simulink model "SingleAgentQUAV"  (R2018b)
settings: Solver=ode1  StartTime=0.0  StopTime=600  FixedStep=tstep  RelTol=1e-3
InitFcn:
  | initSim;
StopFcn:
  | plotSimSolution;
values from neighbouring files (symbols this model uses):
  tstep = 0.1    [initSim.m]
undefined symbols (not defined in the file or in its folder): m, problem
settings Model: Creator=yn15  LastModifiedBy=dan
settings OptimizationCC: LifeSpan=inf
settings DebuggingCC: SFUnexpectedBacktrackingDiag=warning  SFNoUnconditionalDefaultTransitionDiag=warning  SFExecutionAtInitializationDiag=none
settings SFSimCC: SimUseLocalCustomCode=off
settings RTWCC: RTWUseLocalCustomCode=off
settings CodeAppCC: StateflowObjectComments=on
settings GRTTargetCC: TargetLangStandard=C89/C90 (ANSI)
settings ConfigComp: CovMetricSettings=dw  CovHtmlReporting=on  CovSaveCumulativeToWorkspaceVar=on  CovSaveSingleToWorkspaceVar=on  CovExternalEMLEnable=off

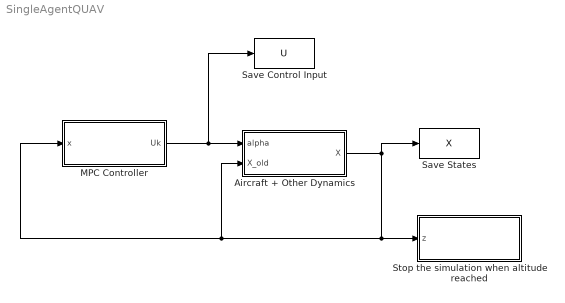
== system SingleAgentQUAV ==
  Aircraft + Other Dynamics : Subsystem
  "MPC Controller " : Subsystem
  Save Control Input : ToWorkspace  VariableName=U  SampleTime=-1
      settings: Save2DSignal=2-D array (concatenate along first dimension)
  Save States : ToWorkspace  VariableName=X  SampleTime=-1
  "Stop the simulation when altitude reached " : Subsystem
  wires:
  "MPC Controller "/1(Uk) -> Aircraft + Other Dynamics/1(alpha), Save Control Input/1
  Aircraft + Other Dynamics/1(X) -> Save States/1, "Stop the simulation when altitude reached "/1(z), Aircraft + Other Dynamics/2("X_old "), "MPC Controller "/1(x)

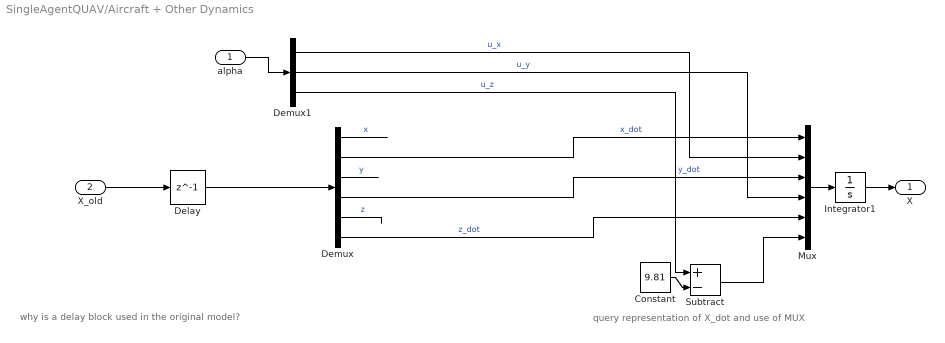
== system SingleAgentQUAV/Aircraft + Other Dynamics ==
  note: query representation of X_dot and use of MUX
  note: why is a delay block used in the original model?
  alpha : Inport
  "X_old " : Inport  Port=2
  Constant : Constant  Value=9.81
  Delay : Delay  DelayLength=1  InitialCondition=[problem.states.x0]
  Demux : Demux  Outputs=6
  Demux1 : Demux  Outputs=3
  Integrator1 : Integrator
  Mux : Mux  Inputs=6
  Subtract : Sum  Inputs=+-
  X : Outport
  wires:
  "X_old "/1 -> Delay/1
  Delay/1 -> Demux/1
  alpha/1 -> Demux1/1
  Demux/1 -> ?  "x"
  Demux/3 -> ?  "y"
  Demux/4 -> Mux/3  "y_dot"
  Demux/5 -> ?  "z"
  Demux/6 -> Mux/5  "z_dot"
  Demux1/1 -> Mux/2  "u_x"
  Demux1/2 -> Mux/4  "u_y"
  Demux1/3 -> Subtract/1  "u_z"
  Demux/2 -> Mux/1  "x_dot"
  Integrator1/1 -> X/1
  Mux/1 -> Integrator1/1
  Constant/1 -> Subtract/2
  Subtract/1 -> Mux/6

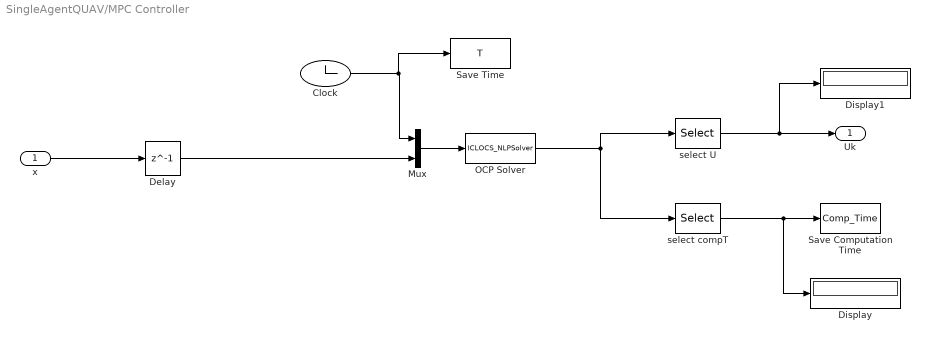
== system SingleAgentQUAV/MPC Controller  ==
  x : Inport
  Clock : Clock
  Delay : Delay  DelayLength=1  InitialCondition=[problem.states.x0]
  Display : Display
  Display1 : Display
  Mux : Mux  Inputs=2
  OCP Solver : MATLABFcn  MATLABFcn=ICLOCS_NLPSolver  OutputDimensions=m+2
  "Save Computation Time " : ToWorkspace  VariableName=Comp_Time  SampleTime=tstep
      settings: Save2DSignal=2-D array (concatenate along first dimension)
  Save Time : ToWorkspace  VariableName=T  SampleTime=-1
      settings: Save2DSignal=2-D array (concatenate along first dimension)
  select U : Selector  IndexOptions=Index vector (dialog)  Indices=3:m+2  OutputSizes=1
  select compT : Selector  IndexOptions=Index vector (dialog)  Indices=2  OutputSizes=1
  Uk : Outport
  wires:
  select U/1 -> Display1/1, Uk/1
  x/1 -> Delay/1
  OCP Solver/1 -> select compT/1, select U/1
  Clock/1 -> Save Time/1, Mux/1
  Mux/1 -> OCP Solver/1
  Delay/1 -> Mux/2
  select compT/1 -> Display/1, "Save Computation Time "/1

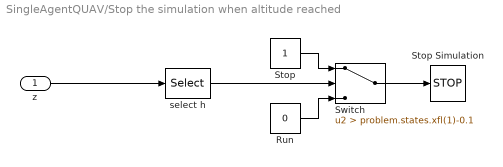
== system SingleAgentQUAV/Stop the simulation when altitude reached  ==
  z : Inport
  Run : Constant  Value=0
  Stop : Constant
  Stop Simulation : Stop
  Switch : Switch  Criteria=u2 > Threshold  Threshold=problem.states.xfl(1)-0.1
  select h : Selector  IndexOptions=Index vector (dialog)  Indices=1  OutputSizes=1
  wires:
  Switch/1 -> Stop Simulation/1
  z/1 -> select h/1
  Stop/1 -> Switch/1
  Run/1 -> Switch/3
  select h/1 -> Switch/2
